simulink model "Test01_SIG"  (Simulink 5.1)
settings: Solver=ode4  StartTime=0.0  StopTime=TMax  FixedStep=DT  MaxStep=DT  RelTol=1e-3
values from neighbouring files (symbols this model uses):
  GBRatio = 22.5    [Run_Test01_SIG.m]
  GenEff = 100.0    (= 100)    [Run_Test01_SIG.m]
  SIG_POTq = SIG_RtTq*SIG_PORt    (= 2735.8)    [Run_Test01_SIG.m]
  SIG_Slop = SIG_RtTq/(SIG_RtSp - SIG_SySp)    (= 719.696022001)    [Run_Test01_SIG.m]
  SIG_SySp = SIG_SySp*pi/30    (= 125.663706144)    [Run_Test01_SIG.m]
undefined symbols (not defined in the file or in its folder): NDOF, NumBl, NumOuts, OutList, q_init, qdot_init, strmatch
libraries: simulink x4
settings Model: LastModifiedBy=jjonkman  SaveTime=off  SaveOutput=off  LimitDataPoints=off  BooleanDataType=on  ProdHWDeviceType=Microprocessor

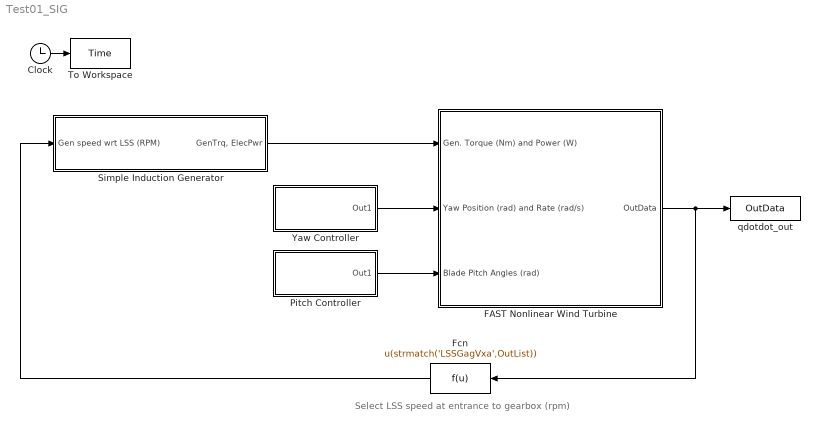
== system Test01_SIG ==
  note: Select LSS speed at entrance to gearbox (rpm)
  Clock : Clock
      settings: Decimation=10
  FAST Nonlinear Wind Turbine : Subsystem  mask(FAST Nonlinear Wind Turbine){}
      mask help: This block contains the FAST S-Function and blocks that integrate the DOF accelerations to get velocities and displacements.
      mask init:
      | clear FAST_SFunc
  Fcn : Fcn  Orientation=left  Expr=u(strmatch('LSSGagVxa',OutList))
  Pitch Controller : Subsystem
  Simple Induction Generator : Subsystem
  To Workspace : ToWorkspace  VariableName=Time  SampleTime=-1  SaveFormat=Array
  Yaw Controller : Subsystem
  qdotdot_out : ToWorkspace  VariableName=OutData  SampleTime=-1  SaveFormat=Array
  wires:
  Clock/1 -> To Workspace/1
  FAST Nonlinear Wind Turbine/1(OutData) -> qdotdot_out/1, Fcn/1
  Simple Induction Generator/1("GenTrq, ElecPwr") -> FAST Nonlinear Wind Turbine/1(Gen. Torque (Nm) and Power (W))
  Yaw Controller/1(Out1) -> FAST Nonlinear Wind Turbine/2(Yaw Position (rad) and Rate (rad/s))
  Pitch Controller/1(Out1) -> FAST Nonlinear Wind Turbine/3(Blade Pitch Angles (rad))
  Fcn/1 -> Simple Induction Generator/1(Gen speed wrt LSS (RPM))

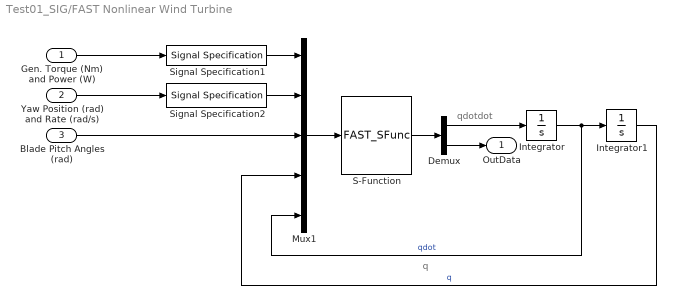
== system Test01_SIG/FAST Nonlinear Wind Turbine ==
  note: qdotdot
  note: q
  Gen. Torque (Nm) and Power (W) : Inport
  Yaw Position (rad) and Rate (rad/s) : Inport  Port=2
  Blade Pitch Angles (rad) : Inport  Port=3
  Demux : Demux  Outputs=[NDOF, NumOuts]
  Integrator : Integrator  InitialCondition=qdot_init
  Integrator1 : Integrator  InitialCondition=q_init
  Mux1 : Mux  Inputs=5
  S-Function : S-Function  FunctionName=FAST_SFunc
  Signal Specification1 : simulink/Signal Attributes/Signal Specification  D=2  Ts=-1  DataType=double  OutDataType=sfix(16)  OutScaling=2^0
      settings: SamplingMode=auto
  Signal Specification2 : simulink/Signal Attributes/Signal Specification  D=2  Ts=-1  DataType=double  OutDataType=sfix(16)  OutScaling=2^0
      settings: SamplingMode=auto
  OutData : Outport
  wires:
  Integrator/1 -> Integrator1/1, Mux1/5  "qdot"
  Gen. Torque (Nm) and Power (W)/1 -> Signal Specification1/1
  S-Function/1 -> Demux/1
  Demux/1 -> Integrator/1
  Demux/2 -> OutData/1
  Mux1/1 -> S-Function/1
  Blade Pitch Angles (rad)/1 -> Mux1/3
  Yaw Position (rad) and Rate (rad/s)/1 -> Signal Specification2/1
  Integrator1/1 -> Mux1/4  "q"
  Signal Specification1/1 -> Mux1/1
  Signal Specification2/1 -> Mux1/2

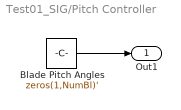
== system Test01_SIG/Pitch Controller ==
  Blade Pitch Angles : Constant  Value=zeros(1,NumBl)'
  Out1 : Outport
  wires:
  Blade Pitch Angles/1 -> Out1/1

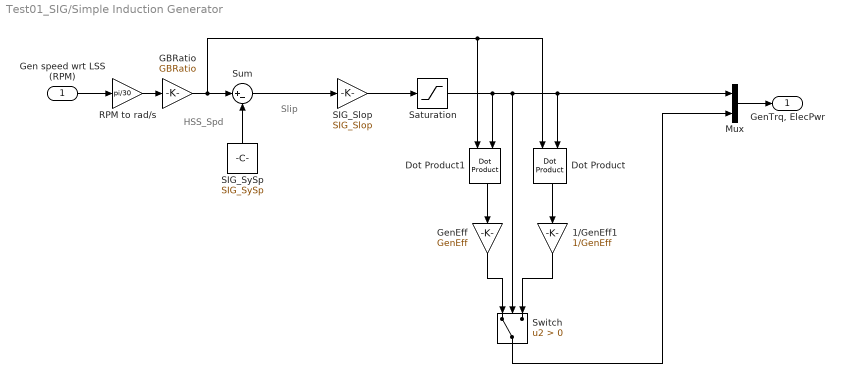
== system Test01_SIG/Simple Induction Generator ==
  note: HSS_Spd
  note: Slip
  Gen speed wrt LSS (RPM) : Inport
  1/GenEff1 : Gain  Orientation=down  Gain=1/GenEff  SaturateOnIntegerOverflow=on
  Dot Product : simulink/Math Operations/Dot Product  Orientation=down
  Dot Product1 : simulink/Math Operations/Dot Product  Orientation=down
  GBRatio : Gain  Gain=GBRatio  SaturateOnIntegerOverflow=on
  GenEff : Gain  Orientation=down  Gain=GenEff  SaturateOnIntegerOverflow=on
  Mux : Mux  Inputs=2
  RPM to rad/s : Gain  Gain=pi/30  SaturateOnIntegerOverflow=on
  SIG_Slop : Gain  Gain=SIG_Slop  SaturateOnIntegerOverflow=on
  SIG_SySp : Constant  Orientation=up  Value=SIG_SySp
  Saturation : Saturate  UpperLimit=SIG_POTq  LowerLimit=-(SIG_POTq)
  Sum : Sum  Inputs=|+-  SaturateOnIntegerOverflow=on
  Switch : Switch  Orientation=down  Criteria=u2 > Threshold  SaturateOnIntegerOverflow=on
  "GenTrq, ElecPwr" : Outport
  wires:
  SIG_SySp/1 -> Sum/2
  GBRatio/1 -> Sum/1, Dot Product/1, Dot Product1/1
  Sum/1 -> SIG_Slop/1
  SIG_Slop/1 -> Saturation/1
  Dot Product/1 -> 1/GenEff1/1
  1/GenEff1/1 -> Switch/3
  GenEff/1 -> Switch/1
  Dot Product1/1 -> GenEff/1
  Saturation/1 -> Dot Product1/2, Dot Product/2, Mux/1, Switch/2
  Mux/1 -> "GenTrq, ElecPwr"/1
  RPM to rad/s/1 -> GBRatio/1
  Switch/1 -> Mux/2
  Gen speed wrt LSS (RPM)/1 -> RPM to rad/s/1

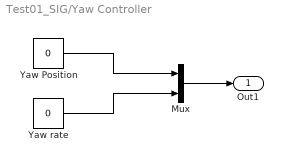
== system Test01_SIG/Yaw Controller ==
  Mux : Mux  Inputs=2
  Yaw Position : Constant  Value=0
  Yaw rate : Constant  Value=0
  Out1 : Outport
  wires:
  Mux/1 -> Out1/1
  Yaw Position/1 -> Mux/1
  Yaw rate/1 -> Mux/2
